simulink model "Target_Control_System"  (R2021b)
settings: Solver=FixedStepDiscrete  StartTime=0.0  StopTime=5  RelTol=1e-3
PreLoadFcn:
  | RTWConfigurationCB('preloadfcn', bdroot);
PostLoadFcn:
  | load('configuration/data_struct.mat');
  | load('configuration/fluxMaps_propMotor.mat');
  | load('configuration/parameterInit_PROP.mat');
  | load('configuration/parameterInit_PUMP.mat');
  | load('configuration/parameterInit_PITCH.mat');
  | load('configuration/parameterInit_TILT.mat');
  | %load('configuration/base_workspace_signal_definition.mat');
  | %load('resolvedatastores_to_baseworkspace_for_faster_simulation.mat');
model workspace (MAT data in the model file):
  SIMULATION_OPTIONS : Simulink.Parameter (value not decoded)
  TARGET_CODE_GEN : Simulink.Parameter (value not decoded)
  TCS_SAMPLE_FREQ_HZ : Simulink.Parameter (value not decoded)
symbols that are objects in the model workspace (value not decoded): TARGET_CODE_GEN, TCS_SAMPLE_FREQ_HZ
undefined symbols (not defined in the file): A_DQ_REF_LPF_INIT__PITCH, A_DQ_REF_LPF_INIT__PROP, A_DQ_REF_LPF_INIT__PUMP, A_DQ_REF_LPF_INIT__TILT, A_OBSERVER_CONFIDENCE_INIT__PITCH, A_OBSERVER_CONFIDENCE_INIT__PROP, A_OBSERVER_CONFIDENCE_INIT__PUMP, A_OBSERVER_CONFIDENCE_INIT__TILT, ACTUATOR_MAX_ANGLE_TRIP__PITCH, ACTUATOR_MIN_ANGLE_TRIP__PITCH, ACTUATOR_POS_SENSOR_INV_DIRECTION__PITCH, ACTUATOR_POS_SENSOR_INV_DIRECTION__TILT, ACTUATOR_POS_SENSOR_OFFSET__PITCH, ACTUATOR_POS_SENSOR_OFFSET__TILT, ADC_scaler1_baseaddr_TILT, ADC_SCALER_FLOAT_TO_FIXPOINT_EXPANSION, ANGLE_ELEC_FROM_SENSOR_OFFSET_INIT__PITCH, ANGLE_ELEC_FROM_SENSOR_OFFSET_INIT__PROP, ANGLE_ELEC_FROM_SENSOR_OFFSET_INIT__PUMP, ANGLE_ELEC_FROM_SENSOR_OFFSET_INIT__TILT, AUTO_CLEAR_FAULTS_ENABLED__PITCH, AUTO_CLEAR_FAULTS_ENABLED__PROP, AUTO_CLEAR_FAULTS_ENABLED__PUMP, AUTO_CLEAR_FAULTS_ENABLED__TILT, AUTO_CLEAR_FAULTS_WAIT_TICKS__PITCH, AUTO_CLEAR_FAULTS_WAIT_TICKS__PROP, AUTO_CLEAR_FAULTS_WAIT_TICKS__PUMP, AUTO_CLEAR_FAULTS_WAIT_TICKS__TILT, AUTO_I_ZERO_IDLE_TICKS__PITCH, AUTO_I_ZERO_IDLE_TICKS__PROP, AUTO_I_ZERO_IDLE_TICKS__PUMP, AUTO_I_ZERO_IDLE_TICKS__TILT, AUTO_I_ZERO_OFFSET_IDC_THRESHOLD__PITCH, AUTO_I_ZERO_OFFSET_IDC_THRESHOLD__PROP, AUTO_I_ZERO_OFFSET_IDC_THRESHOLD__PUMP, AUTO_I_ZERO_OFFSET_IDC_THRESHOLD__TILT, AUTO_I_ZERO_OFFSET_IPH_THRESHOLD__PITCH, AUTO_I_ZERO_OFFSET_IPH_THRESHOLD__PROP, AUTO_I_ZERO_OFFSET_IPH_THRESHOLD__PUMP, AUTO_I_ZERO_OFFSET_IPH_THRESHOLD__TILT, AUTO_SENSORLESS_SWITCHOVER_DISABLE_OMEGA, AUTO_SENSORLESS_SWITCHOVER_ENABLE_OMEGA, AUTO_SENSORLESS_SWITCHOVER_MIN_CONFIDENCE, AUXILIARY_PROTECTION_UNIT_BASEADDR__TILT, blanking_max_error_omega_INIT_PITCH, blanking_max_error_omega_INIT_TILT, blanking_max_error_position_INIT_PITCH, blanking_max_error_position_INIT_TILT, BRUTE_START_I_Q_REF_RAMP_SPEED__PITCH, BRUTE_START_I_Q_REF_RAMP_SPEED__PROP, BRUTE_START_I_Q_REF_RAMP_SPEED__PUMP, BRUTE_START_I_Q_REF_RAMP_SPEED__TILT, CONTROL_LOOP_DT_INIT__PITCH, CONTROL_LOOP_DT_INIT__PROP, CONTROL_LOOP_DT_INIT__PUMP, CONTROL_LOOP_DT_INIT__TILT, CORRECTION_FILTER_SCALE__PITCH, CORRECTION_FILTER_SCALE__PROP, CORRECTION_FILTER_SCALE__PUMP, CORRECTION_FILTER_SCALE__TILT ... (+458)
libraries: simulink x178, Reusables_Lib x24
(part 46 of 47)

== stateflow chart Target_Control_System/InterruptFunction/propMotor_isrTask/isrStateMachine/ISR State Machine ==
  state SuperState
    state ISR_States [parallel]
      // Main drive not active, just idle or various auxiliary operating modes
      // Do specific things:
      settings: executionOrder=3
      state Start
      state initiateCurrentOffsetNulling
        during:
        //Run an I controller for each current channel to be zerod, that zeros the actual reading
        // Note: the address to write out to
        oProp.oIsr_.oState_.fOffsetIntegratorIa_ += oProp.oIsr_.oIn_.oAdcData_.fIa_;
        oProp.oIsr_.oOut_.iOffsetIa_ -= cast((500.0F*oProp.oIsr_.oIn_.oAdcData_.fIa_ + 0.01F*oProp.oIsr_.oState_.fOffsetIntegratorIa_), int32);
        oProp.oIsr_.oState_.fOffsetIntegratorIb_ += oProp.oIsr_.oIn_.oAdcData_.fIb_;
        oProp.oIsr_.oOut_.iOffsetIb_ -= cast((500.0F*oProp.oIsr_.oIn_.oAdcData_.fIb_ + 0.01F*oProp.oIsr_.oState_.fOffsetIntegratorIb_), int32);
        oProp.oIsr_.oState_.fOffsetIntegratorIc_ += oProp.oIsr_.oIn_.oAdcData_.fIc_;
        oProp.oIsr_.oOut_.iOffsetIc_ -= cast((500.0F*oProp.oIsr_.oIn_.oAdcData_.fIc_ + 0.01F*oProp.oIsr_.oState_.fOffsetIntegratorIc_), int32);
        oProp.oIsr_.oState_.fOffsetIntegratorIdc_ += oProp.oIsr_.oIn_.oAdcData_.fIdc_;
        oProp.oIsr_.oOut_.iOffsetIdc_ -= cast((500.0F*oProp.oIsr_.oIn_.oAdcData_.fIdc_ + 0.01F*oProp.oIsr_.oState_.fOffsetIntegratorIdc_), int32);
        oProp.oIsr_.oOut_.iIBiasUpdated_ = 1;
      state CaptureAverageVoltage
        during:
        //At 50% duty, capture intended average phase voltage
        oProp.oIsr_.oState_.fOffsetAvgUphase_ += 0.001F * (oProp.oIsr_.oIn_.oAdcData_.fUdc_ * 0.5F - oProp.oIsr_.oState_.fOffsetAvgUphase_);
      state initiateVoltageOffsetNulling
        during:
        // At 50% duty, zero the voltage to the average voltage
        fTemp = oProp.oIsr_.oIn_.oAdcData_.fUa_ - oProp.oIsr_.oState_.fOffsetAvgUphase_;
        oProp.oIsr_.oState_.fOffsetIntegratorUa_ += fTemp;
        oProp.oIsr_.oOut_.iOffsetUa_ -= cast((50.0F * fTemp + 0.02F * oProp.oIsr_.oState_.fOffsetIntegratorUa_), int32);
        fTemp = oProp.oIsr_.oIn_.oAdcData_.fUb_ - oProp.oIsr_.oState_.fOffsetAvgUphase_;
        oProp.oIsr_.oState_.fOffsetIntegratorUb_ += fTemp;
        oProp.oIsr_.oOut_.iOffsetUb_ -= cast((50.0F * fTemp + 0.01F * oProp.oIsr_.oState_.fOffsetIntegratorUb_), int32);
        fTemp = oProp.oIsr_.oIn_.oAdcData_.fUc_ - oProp.oIsr_.oState_.fOffsetAvgUphase_;
        oProp.oIsr_.oState_.fOffsetIntegratorUc_ += fTemp;
        oProp.oIsr_.oOut_.iOffsetUc_ -= cast((50.0F * fTemp + 0.005F * oProp.oIsr_.oState_.fOffsetIntegratorUc_), int32);
        oProp.oIsr_.oOut_.iUBiasUpdated_ = 1;
      (default) -> Start
      Start -> initiateCurrentOffsetNulling [order 1] : [oProp.oIsr_.oIn_.uiDriveState_ == 95]
      initiateCurrentOffsetNulling -> Start : [!(oProp.oIsr_.oIn_.uiDriveState_ == 95)]
      Start -> CaptureAverageVoltage [order 2] : [oProp.oIsr_.oIn_.uiDriveState_ == 250 || oProp.oIsr_.oIn_.uiDriveState_ == 245]
      CaptureAverageVoltage -> Start : [!(oProp.oIsr_.oIn_.uiDriveState_ == 250 || oProp.oIsr_.oIn_.uiDriveState_ == 245)]
      Start -> initiateVoltageOffsetNulling [order 3] : [oProp.oIsr_.oIn_.uiDriveState_ == 251 || oProp.oIsr_.oIn_.uiDriveState_ == 246]
      initiateVoltageOffsetNulling -> Start : [!(oProp.oIsr_.oIn_.uiDriveState_ == 251 || oProp.oIsr_.oIn_.uiDriveState_ == 246)]
    state Software_overcurrent_protection [parallel]
      settings: executionOrder=2
      state Nominal
      state Fault
        state Fault_A
          entry:
          oProp.oMot_.oOut_.uiCurrentControllerActive_ = 0;
          oProp.oMot_.oOut_.uiEnableGateDrive_ = 0;
        state Fault_B
          // If we were already in a fault state, store the previous fault:
          entry:
          oProp.oMot_.oOut_.uiLastFaultState_ = oProp.oMot_.oState_.uiDriveState_;
        state Fault_C
          entry:
          oProp.oMot_.oState_.uiDriveState_ = 1007;
        (default) -> (junction 153)
        (junction 153) -> Fault_C [order 3]
        (junction 153) -> Fault_B [order 2] : [oProp.oMot_.oState_.uiDriveState_>= 1000]
        (junction 153) -> Fault_A [order 1] : [oProp.oMot_.oState_.uiDriveState_>= 200]
        Fault_A -> Fault_C [order 2]
        Fault_A -> Fault_B [order 1] : [oProp.oMot_.oState_.uiDriveState_>= 1000]
        Fault_B -> Fault_C
      (default) -> Nominal
      Fault -> Nominal : [oProp.oIsr_.oOut_.fIPhaseMagnitude_<oProp.oMot_.oParam_.fTripLimitSoftwareA_]
      Nominal -> Fault : [oProp.oIsr_.oOut_.fIPhaseMagnitude_>oProp.oMot_.oParam_.fTripLimitSoftwareA_]
    state Forced_Angle_State_Manager [parallel]
      settings: executionOrder=1
      state InitialForcedAngleState
        during:
        oProp.oMot_.oState_.oRampDataFluxMstrAngFrcd2clsdSmoothn_.fRampOut_ = 0.0F;
      state ForcedAngleState
        entry:
        oProp.oMot_.oOut_.uiForcedAngle_ = 1;
        during:
        oProp.oMot_.oState_.oRampDataFluxMstrAngFrcd2clsdSmoothn_.fRampOut_ = oProp.oIsr_.oState_.fFluxMasterAngle_ - oProp.oIsr_.oState_.fFluxMainAngleRaw2_;
      (default) -> InitialForcedAngleState
      InitialForcedAngleState -> ForcedAngleState : [oProp.oMot_.oState_.uiDriveState_ == 211 || oProp.oMot_.oState_.uiDriveState_ == 212]
      ForcedAngleState -> InitialForcedAngleState : [!(oProp.oMot_.oState_.uiDriveState_ == 211 || oProp.oMot_.oState_.uiDriveState_ == 212)]{oProp.oMot_.oOut_.uiForcedAngle_ = 0;}
  (default) -> SuperState
  data: oProp data_store_memory; fTemp local single

== stateflow chart Target_Control_System/InterruptFunction/pumpMotor_isrTask/isrStateMachine/ISR State Machine ==
  state SuperState
    state ISR_States [parallel]
      // Main drive not active, just idle or various auxiliary operating modes
      // Do specific things:
      settings: executionOrder=3
      state Start
      state initiateOffsetNulling
        during:
        //Run an I controller for each current channel to be zerod, that zeros the actual reading
        // Note: the address to write out to
        oPump.oIsr_.oState_.fOffsetIntegratorIa_ += oPump.oIsr_.oIn_.oAdcData_.fIa_;
        oPump.oIsr_.oOut_.iOffsetIa_ -= cast((500.0F*oPump.oIsr_.oIn_.oAdcData_.fIa_ + 0.01F*oPump.oIsr_.oState_.fOffsetIntegratorIa_), int32);
        oPump.oIsr_.oState_.fOffsetIntegratorIb_ += oPump.oIsr_.oIn_.oAdcData_.fIb_;
        oPump.oIsr_.oOut_.iOffsetIb_ -= cast((500.0F*oPump.oIsr_.oIn_.oAdcData_.fIb_ + 0.01F*oPump.oIsr_.oState_.fOffsetIntegratorIb_), int32);
        oPump.oIsr_.oState_.fOffsetIntegratorIc_ += oPump.oIsr_.oIn_.oAdcData_.fIc_;
        oPump.oIsr_.oOut_.iOffsetIc_ -= cast((500.0F*oPump.oIsr_.oIn_.oAdcData_.fIc_ + 0.01F*oPump.oIsr_.oState_.fOffsetIntegratorIc_), int32);
        oPump.oIsr_.oState_.fOffsetIntegratorIdc_ += oPump.oIsr_.oIn_.oAdcData_.fIdc_;
        oPump.oIsr_.oOut_.iOffsetIdc_ -= cast((500.0F*oPump.oIsr_.oIn_.oAdcData_.fIdc_ + 0.01F*oPump.oIsr_.oState_.fOffsetIntegratorIdc_), int32);
        oPump.oIsr_.oOut_.iIBiasUpdated_ = 1;
      (default) -> Start
      Start -> initiateOffsetNulling : [oPump.oMot_.oState_.uiDriveState_ == 95]
      initiateOffsetNulling -> Start : [!(oPump.oMot_.oState_.uiDriveState_ == 95)]
    state Forced_Angle_State_Manager [parallel]
      settings: executionOrder=1
      state InitialForcedAngleState
        during:
        oPump.oMot_.oState_.oRampDataFluxMstrAngFrcd2clsdSmoothn_.fRampOut_ = 0;
      state ForcedAngleState
        entry:
        oPump.oMot_.oOut_.uiForcedAngle_ = 1;
        during:
        oPump.oMot_.oState_.oRampDataFluxMstrAngFrcd2clsdSmoothn_.fRampOut_ = oPump.oIsr_.oState_.fFluxMasterAngle_ - oPump.oIsr_.oState_.fFluxMainAngleRaw2_;
      (default) -> InitialForcedAngleState
      InitialForcedAngleState -> ForcedAngleState : [oPump.oMot_.oState_.uiDriveState_ == 211 || oPump.oMot_.oState_.uiDriveState_ == 212]
      ForcedAngleState -> InitialForcedAngleState : [!(oPump.oMot_.oState_.uiDriveState_ == 211 || oPump.oMot_.oState_.uiDriveState_ == 212)]{oPump.oMot_.oOut_.uiForcedAngle_ = 0;}
    state Software_overcurrent_protection [parallel]
      settings: executionOrder=2
      state Nominal
      state Fault
        state Fault_A
          entry:
          oPump.oMot_.oOut_.uiCurrentControllerActive_ = 0;
          oPump.oMot_.oOut_.uiEnableGateDrive_ = 0;
        state Fault_B
          // If we were already in a fault state, store the previous fault:
          entry:
          oPump.oMot_.oOut_.uiLastFaultState_ = oPump.oMot_.oState_.uiDriveState_;
        state Fault_C
          entry:
          oPump.oMot_.oState_.uiDriveState_ = 1007;
        (default) -> (junction 153)
        (junction 153) -> Fault_C [order 3]
        (junction 153) -> Fault_B [order 2] : [oPump.oMot_.oState_.uiDriveState_>= 1000]
        (junction 153) -> Fault_A [order 1] : [oPump.oMot_.oState_.uiDriveState_>= 200]
        Fault_A -> Fault_C [order 2]
        Fault_A -> Fault_B [order 1] : [oPump.oMot_.oState_.uiDriveState_>= 1000]
        Fault_B -> Fault_C
      (default) -> Nominal
      Fault -> Nominal : [oPump.oIsr_.oOut_.fIPhaseMagnitude_<oPump.oMot_.oParam_.fTripLimitSoftwareA_]
      Nominal -> Fault : [oPump.oIsr_.oOut_.fIPhaseMagnitude_>oPump.oMot_.oParam_.fTripLimitSoftwareA_]
  (default) -> SuperState
  data: oPump data_store_memory

== stateflow chart Target_Control_System/InterruptFunction/tiltMotor_isrTask/isrStateMachine/ISR State Machine ==
  state SuperState
    state ISR_States [parallel]
      // Main drive not active, just idle or various auxiliary operating modes
      // Do specific things:
      settings: executionOrder=1
      state Start
      state initiateCurrentOffsetNulling
        during:
        //Run an I controller for each current channel to be zerod, that zeros the actual reading
        // Note: the address to write out to
        oTilt.oIsr_.oState_.fOffsetIntegratorIa_ += oTilt.oIsr_.oIn_.oAdcData_.fIa_;
        oTilt.oIsr_.oOut_.iOffsetIa_ -= cast((500.0F*oTilt.oIsr_.oIn_.oAdcData_.fIa_ + 0.01F*oTilt.oIsr_.oState_.fOffsetIntegratorIa_), int32);
        oTilt.oIsr_.oState_.fOffsetIntegratorIb_ += oTilt.oIsr_.oIn_.oAdcData_.fIb_;
        oTilt.oIsr_.oOut_.iOffsetIb_ -= cast((500.0F*oTilt.oIsr_.oIn_.oAdcData_.fIb_ + 0.01F*oTilt.oIsr_.oState_.fOffsetIntegratorIb_), int32);
        oTilt.oIsr_.oState_.fOffsetIntegratorIc_ += oTilt.oIsr_.oIn_.oAdcData_.fIc_;
        oTilt.oIsr_.oOut_.iOffsetIc_ -= cast((500.0F*oTilt.oIsr_.oIn_.oAdcData_.fIc_ + 0.01F*oTilt.oIsr_.oState_.fOffsetIntegratorIc_), int32);
        oTilt.oIsr_.oState_.fOffsetIntegratorIdc_ += oTilt.oIsr_.oIn_.oAdcData_.fIdc_;
        oTilt.oIsr_.oOut_.iOffsetIdc_ -= cast((500.0F*oTilt.oIsr_.oIn_.oAdcData_.fIdc_ + 0.01F*oTilt.oIsr_.oState_.fOffsetIntegratorIdc_), int32);
        oTilt.oIsr_.oOut_.iIBiasUpdated_ = 1;
      state CaptureAverageVoltage
        during:
        //At 50% duty, capture intended average phase voltage
        oTilt.oIsr_.oState_.fOffsetAvgUphase_ += 0.001F * (oTilt.oIsr_.oIn_.oAdcData_.fUdc_ * 0.5F - oTilt.oIsr_.oState_.fOffsetAvgUphase_);
      state initiateVoltageOffsetNulling
        during:
        // At 50% duty, zero the voltage to the average voltage
        fTemp = oTilt.oIsr_.oIn_.oAdcData_.fUa_ - oTilt.oIsr_.oState_.fOffsetAvgUphase_;
        oTilt.oIsr_.oState_.fOffsetIntegratorUa_ += fTemp;
        oTilt.oIsr_.oOut_.iOffsetUa_ -= cast((50.0F * fTemp + 0.02F * oTilt.oIsr_.oState_.fOffsetIntegratorUa_), int32);
        fTemp = oTilt.oIsr_.oIn_.oAdcData_.fUb_ - oTilt.oIsr_.oState_.fOffsetAvgUphase_;
        oTilt.oIsr_.oState_.fOffsetIntegratorUb_ += fTemp;
        oTilt.oIsr_.oOut_.iOffsetUb_ -= cast((50.0F * fTemp + 0.01F * oTilt.oIsr_.oState_.fOffsetIntegratorUb_), int32);
        fTemp = oTilt.oIsr_.oIn_.oAdcData_.fUc_ - oTilt.oIsr_.oState_.fOffsetAvgUphase_;
        oTilt.oIsr_.oState_.fOffsetIntegratorUc_ += fTemp;
        oTilt.oIsr_.oOut_.iOffsetUc_ -= cast((50.0F * fTemp + 0.005F * oTilt.oIsr_.oState_.fOffsetIntegratorUc_), int32);
        oTilt.oIsr_.oOut_.iUBiasUpdated_ = 1;
      (default) -> Start
      Start -> initiateCurrentOffsetNulling [order 1] : [oTilt.oIsr_.oIn_.uiDriveState_ == 95]
      initiateCurrentOffsetNulling -> Start : [!(oTilt.oIsr_.oIn_.uiDriveState_ == 95)]
      Start -> CaptureAverageVoltage [order 2] : [oTilt.oIsr_.oIn_.uiDriveState_ == 250 || oTilt.oIsr_.oIn_.uiDriveState_ == 245]
      CaptureAverageVoltage -> Start : [!(oTilt.oIsr_.oIn_.uiDriveState_ == 250 || oTilt.oIsr_.oIn_.uiDriveState_ == 245)]
      Start -> initiateVoltageOffsetNulling [order 3] : [oTilt.oIsr_.oIn_.uiDriveState_ == 251 || oTilt.oIsr_.oIn_.uiDriveState_ == 246]
      initiateVoltageOffsetNulling -> Start : [!(oTilt.oIsr_.oIn_.uiDriveState_ == 251 || oTilt.oIsr_.oIn_.uiDriveState_ == 246)]
  (default) -> SuperState
  data: oTilt data_store_memory; fTemp local single

== stateflow chart Target_Control_System/MainLoop/tiltMotor_mainLoop/Decimation gate for 200 Hz Tilt/motorTaskMainDecimationAStep(&oTilt)/Check zero current if inverter off/Enabled Subsystem/Chart ==
  state Start
  state Drive_trip
    // Disable the drive and enter a trip state (error state)
    entry:
    oTilt.oMot_.oOut_.uiEnableGateDrive_ = 0;
    oTilt.oMot_.oOut_.uiCurrentControllerActive_ = 0;
    // NOTE: the actual turning off is done in the ctrl interrupt
    // formerly: Xil_Out32(uiGateDriverBaseaddr_, 0x0);
  state Store_previous_fault
    // If we were already in a fault state, store the previous fault:
    entry:
    oTilt.oMot_.oOut_.uiLastFaultState_ = oTilt.oMot_.oState_.uiDriveState_;
  state setTripState
    entry:
    oTilt.oMot_.oState_.uiDriveState_ = 1042;
  (default) -> Start
  setTripState -> Start
  Start -> (junction 14) : [fabs(oTilt.oMot_.oIn_.oAdcData_.fIa_) > oTilt.oMot_.oParam_.fMaximumPhaseCurrentWhileOff_ || ...
      | fabs(oTilt.oMot_.oIn_.oAdcData_.fIb_) > oTilt.oMot_.oParam_.fMaximumPhaseCurrentWhileOff_ || ...
      | fabs(oTilt.oMot_.oIn_.oAdcData_.fIc_) > oTilt.oMot_.oParam_.fMaximumPhaseCurrentWhileOff_]
  (junction 14) -> Drive_trip [order 1] : [oTilt.oMot_.oState_.uiDriveState_ >= 200]
  (junction 14) -> (junction 19) [order 2]
  Drive_trip -> (junction 19)
  (junction 19) -> Store_previous_fault [order 1] : [oTilt.oMot_.oState_.uiDriveState_ >= 1000]
  (junction 19) -> setTripState [order 2]
  Store_previous_fault -> setTripState
  data: oTilt data_store_memory

== stateflow chart Target_Control_System/MainLoop/propMotor_mainLoop/motorStateMachineLogic(&oProp)/Idle-Loop State Machine Prop ==
  state motorStateMachineLogic
  state State_90
    //startup delay
    state Wait_Ticks_
    state Startup_Delay_
      entry:
      oProp.oMot_.oState_.uiDriveState_ = 95;
      oProp.oMot_.oOut_.uiLastFaultState_ = 0;
    (default) -> State_90.Wait_Ticks_
    State_90.Wait_Ticks_ -> Startup_Delay_ : [after(35, tick)]
  state State_246
    // Second phase of voltage nulling
    state Wait_uiDelayTicks_
    state Next
      entry:
      oProp.oMot_.oState_.uiDriveState_ = 100;
      oProp.oMot_.oOut_.uiEnableGateDrive_ = 0x0;
      oProp.oMot_.oIn_.uiVoltageOffsetNullingActive_ = 0;
    (default) -> State_246.Wait_uiDelayTicks_
    State_246.Wait_uiDelayTicks_ -> State_246.Next : [after(25, tick)]
  state State_95
    // Current offset nulling
    state Wait_Ticks_
    state Current_offset_nulling
      entry:
      oProp.oMot_.oState_.uiCurrentOffsetNullingPerformed_++;
      oProp.oMot_.oIn_.uiCurrentOffsetNullingActive_ = 0;
      oProp.oMot_.oIn_.uiVoltageOffsetNullingActive_ = 0;
      oProp.oMot_.oState_.uiDriveState_ = 99;
      //SZ: still need to re-write the FPGA protection to enable the sum of current detection for fault 1034
    (default) -> State_95.Wait_Ticks_
    State_95.Wait_Ticks_ -> Current_offset_nulling : [after(6, tick)]
  state State_245
    // Initial phase of voltage nulling
    state Wait_uiDelayTicks_
    state Next
      entry:
      oProp.oMot_.oState_.uiDriveState_ = 246;
    (default) -> State_245.Wait_uiDelayTicks_
    State_245.Wait_uiDelayTicks_ -> State_245.Next : [after(25, tick)]
  state State_99
    // Minimum command set not met. Also the return state after clearing trips etc.
    state Substate
    state Idle_state
      entry:
      oProp.oMot_.oState_.uiDriveState_ = 100;
    state Cleanup
      // We somehow left the forced angle start sequence without cleaning up.
      // Clean up now.
      entry:
      oProp.oMot_.oState_.oRampDataOmegaERef_.oParam_.fUpslope_ = oProp.oMot_.oState_.fForcedAngleStartOrigOmegaRamp_;
      oProp.oMot_.oState_.oRampDataOmegaERef_.fSetpoint_ = fabs(oProp.oMot_.oState_.fForcedAngleStartOrigOmega_);
      oProp.oMot_.oState_.uiSpeedControllerActive_ = oProp.oMot_.oState_.uiForcedAngleStartOrigSpeedControllerActive_;
      oProp.oMot_.oState_.oRampDataIqRef_.oParam_.fUpslope_ = oProp.oMot_.oState_.fForcedAngleStartOrigIRamp_;
      oProp.oMot_.oState_.oRampDataIqRef_.oParam_.fDownslope_ = oProp.oMot_.oState_.oRampDataIqRef_.oParam_.fUpslope_;
      oProp.oMot_.oOut_.uiForcedAngle_ = 0;
      oProp.oMot_.oState_.uiForcedAngleStartParametersSet_ = 0;
    (default) -> State_99.Substate
    State_99.Substate -> (junction 218)
    (junction 218) -> Idle_state [order 2] : [!oProp.oMot_.oState_.uiMinimumCommandSetFlags_]
    (junction 218) -> State_99.Cleanup [order 1] : [oProp.oMot_.oState_.uiForcedAngleStartParametersSet_]
    State_99.Cleanup -> Idle_state : [!oProp.oMot_.oState_.uiMinimumCommandSetFlags_]
  state State_104
    // Idle, motor spinning (windmilling, coasting down),
    // autostart enabled, and a nonzero current applied
    // Removed autostart functionality
    entry:
    oProp.oMot_.oState_.uiDriveState_ = 102;
  state State_103
    // Idle, motor not spinning, autostart enabled, and a nonzero current applied
    // Removed autostart functionality
    entry:
    oProp.oMot_.oState_.uiDriveState_ = 101;
  state State_100
    //Idle, determine if the motor is externally driven (e.g. windmilling or spindown) or standing still
    state Initialization
      entry:
      oProp.oMot_.oState_.oRampDataOmegaERef_.fRampOut_ = 0.0;
      oProp.oMot_.oState_.oRampDataIqRef_.fRampOut_ = 0.0;
    state Entering_State_101
      entry:
      oProp.oMot_.oState_.uiDriveState_ = 101;
    state Cleanup
      // We somehow left the forced angle start sequence without cleaning up.
      // Clean up now.
      entry:
      oProp.oMot_.oState_.uiDriveState_  = 99;
    state Entering_State_102
      entry:
      oProp.oMot_.oState_.uiDriveState_ = 102;
    state pwm50PercentDuty
      //Pre-set 50% duty
      entry:
      oProp.oMot_.oOut_.uiPwmRequestFromMain_ = 1;
      oProp.oMot_.oOut_.uiPwmDutyTicksFromMainA_ = cast(((oProp.oMot_.oParam_.fPwmPeriodTicksMainloopFloat_) / 2), uint32);
      oProp.oMot_.oOut_.uiPwmDutyTicksFromMainB_ = cast(((oProp.oMot_.oParam_.fPwmPeriodTicksMainloopFloat_) / 2), uint32);
      oProp.oMot_.oOut_.uiPwmDutyTicksFromMainC_ = cast(((oProp.oMot_.oParam_.fPwmPeriodTicksMainloopFloat_) / 2), uint32);
    (default) -> State_100.Initialization
    State_100.Initialization -> (junction 235)
    (junction 235) -> (junction 251) [order 2]
    (junction 251) -> Entering_State_101 [order 1] : [(fabs(oProp.oMot_.oOut_.fOmegaEObserverXlpf2_) < oProp.oMot_.oParam_.fFlyingStartOmegaELimit_) ....
        |  || (oProp.oMot_.oState_.fObserverConfidence_ < 0.7F)]
    (junction 235) -> State_100.Cleanup [order 1] : [oProp.oMot_.oState_.uiMinimumCommandSetFlags_]
    (junction 251) -> Entering_State_102 [order 2]
    Entering_State_101 -> pwm50PercentDuty
    Entering_State_102 -> pwm50PercentDuty
  state State_224
    state Transition_220
      // Direction or confidence check failed, restart full sequence
      entry:
      oProp.oMot_.oState_.uiDriveState_ = 220;
    state FlyingStart
      entry:
      oProp.oMot_.oOut_.uiPwmDutyTicksFromMainA_ = uint32((oProp.oMot_.oParam_.fPwmPeriodTicksMainloopFloat_)/2);
      oProp.oMot_.oOut_.uiPwmDutyTicksFromMainB_ = uint32((oProp.oMot_.oParam_.fPwmPeriodTicksMainloopFloat_)/2);
      oProp.oMot_.oOut_.uiPwmDutyTicksFromMainC_ = uint32((oProp.oMot_.oParam_.fPwmPeriodTicksMainloopFloat_)/2);
      oProp.oMot_.oState_.oRampDataOmegaERef_.fRampOut_ = oProp.oMot_.oIn_.fOmegaEObserverLpf2_;
      oProp.oMot_.oState_.oRampDataIqRef_.fRampOut_ = 0.0;
      oProp.oIsr_.oParam_.oPiDataIq_.fState_ = 0.0F;
      oProp.oIsr_.oParam_.oPiDataId_.fState_ = 0.0F;
      oProp.oMot_.oParam_.oPiDataRpm_.fState_ = 0.0F;
      oProp.oMot_.oParam_.oPid2DataRpmCtrl_.fState_ = 0.0F;
      oProp.oMot_.oState_.uiDriveState_ = 200;
      // release gate signals
      oProp.oMot_.oOut_.uiEnableGateDrive_ = 0x7;
      // Release control in main interrupt
      oProp.oMot_.oOut_.uiCurrentControllerActive_ = 1;
    state uiAutomaticFanControlMode_
      entry:
      oProp.oMot_.oState_.uiDriveState_ = 205;
    (default) -> (junction 543)
    (junction 543) -> (junction 546) [order 2]
    (junction 543) -> (junction 545) [order 1] : [oProp.oMot_.oState_.fObserverConfidence_ > oProp.oMot_.oParam_.fSlaveStartMinConfidence_ && ....
        | !(oProp.oMot_.oOut_.fOmegaEObserverXlpf2_ * oProp.oMot_.oState_.fForcedAngleStartDirection_ < 0.0F)]
        | // The faster we go, the further we jump in the sequence
        | // [SZ]: need to investigate implementing the __signbitf() function in Stateflow]
    (junction 546) -> State_224.Transition_220
    (junction 545) -> FlyingStart : //Confidence wise we're good to go, but is the speed high enough?
        | [fabs(oProp.oMot_.oOut_.fOmegaEObserverXlpf2_) > ....
        |  (oProp.oMot_.oParam_.fSlaveStartMinOmegaE_)]
    FlyingStart -> State_224.uiAutomaticFanControlMode_ : [oProp.oMot_.oParam_.uiAutomaticFanControlMode_ == 1]
  state State_102
    // Idle, motor spinning by external means (windmilling, downhill, large inertia, ....)
    state Stay_at_102
      entry:
      oProp.oMot_.oState_.uiDriveState_ = 102;
    state Transition_to_101
      entry:
      oProp.oMot_.oState_.uiDriveState_ = 101;
    (default) -> (junction 349)
    (junction 349) -> Stay_at_102 [order 2]
    (junction 349) -> Transition_to_101 [order 1] : [fabs(oProp.oMot_.oOut_.fOmegaEObserverXlpf2_) < oProp.oMot_.oParam_.fFlyingStartOmegaELimit_ ....
        | || oProp.oMot_.oState_.fObserverConfidence_ < 0.65F]
  state State_222
    state Transition_224
      entry:
      oProp.oMot_.oState_.uiDriveState_ = 224;
    state Transition_223
      entry:
      oProp.oMot_.oState_.uiDriveState_ = 223;
    state Transition_220
      // Direction or confidence check failed, restart full sequence
      entry:
      oProp.oMot_.oState_.uiDriveState_ = 220;
    (default) -> (junction 521)
    (junction 521) -> (junction 518) [order 2]
    (junction 521) -> (junction 512) [order 1] : [oProp.oMot_.oState_.fObserverConfidence_ > oProp.oMot_.oParam_.fSlaveStartMinConfidence_ && ....
        | !(oProp.oMot_.oOut_.fOmegaEObserverXlpf2_ * oProp.oMot_.oState_.fForcedAngleStartDirection_ < 0.0F)]
        | // The faster we go, the further we jump in the sequence
        | // [SZ]: need to investigate implementing the __signbitf() function in Stateflow]
    (junction 518) -> State_222.Transition_220
    (junction 512) -> (junction 519) [order 1]
    (junction 519) -> State_222.Transition_224 : [fabs(oProp.oMot_.oOut_.fOmegaEObserverXlpf2_) >....
        |  (oProp.oMot_.oParam_.fSlaveStartMinOmegaE_)]
    (junction 512) -> State_222.Transition_223 [order 2]
  state State_223
    state Transition_220
      // Direction or confidence check failed, restart full sequence
      entry:
      oProp.oMot_.oState_.uiDriveState_ = 220;
    state Transition_224
      entry:
      oProp.oMot_.oState_.uiDriveState_ = 224;
    (default) -> (junction 528)
    (junction 528) -> (junction 524) [order 2]
    (junction 528) -> (junction 533) [order 1] : [oProp.oMot_.oState_.fObserverConfidence_ > oProp.oMot_.oParam_.fSlaveStartMinConfidence_ && ....
        | !(oProp.oMot_.oOut_.fOmegaEObserverXlpf2_ * oProp.oMot_.oState_.fForcedAngleStartDirection_ < 0.0F)]
        | // The faster we go, the further we jump in the sequence
        | // [SZ]: need to investigate implementing the __signbitf() function in Stateflow]
    (junction 524) -> State_223.Transition_220
    (junction 533) -> State_223.Transition_224 : [fabs( oProp.oMot_.oOut_.fOmegaEObserverXlpf2_) >....
        |  (oProp.oMot_.oParam_.fSlaveStartMinOmegaE_)]
  state State_101
    // Idle, motor not spinning
    state Initialization
      entry:
      oProp.oMot_.oState_.oRampDataOmegaERef_.fRampOut_ = 0.0;
      oProp.oMot_.oState_.oRampDataIqRef_.fRampOut_ = 0.0;
    state Transition_to_102
      entry:
      oProp.oMot_.oState_.uiDriveState_ = 102;
    (default) -> State_101.Initialization
    State_101.Initialization -> (junction 340)
    (junction 340) -> Transition_to_102 [order 1] : [(fabs(oProp.oMot_.oOut_.fOmegaEObserverXlpf2_) > oProp.oMot_.oParam_.fFlyingStartOmegaELimit_) ....
        | && (oProp.oMot_.oState_.fObserverConfidence_ > 0.65F)]
  state State_220
    // Flying start, first of multiple stages.
    // There has to be an uninterrupted chain of OKs. Too low confidence at any step,
    // and fall back to this initial state.
    state Substate
    state Transition_224
      entry:
      oProp.oMot_.oState_.uiDriveState_ = 224;
    state Transition_223
      entry:
      oProp.oMot_.oState_.uiDriveState_ = 223;
    state Transition_222
      entry:
      oProp.oMot_.oState_.uiDriveState_ = 222;
    state Transition_221
      /* Don't check for the speed for the slowest
      //advancement path, that will happen in state 224 */
      entry:
      oProp.oMot_.oState_.uiDriveState_ = 221;
    (default) -> State_220.Substate
    State_220.Substate -> (junction 443)
    (junction 443) -> (junction 396) : [oProp.oMot_.oState_.fObserverConfidence_ > oProp.oMot_.oParam_.fSlaveStartMinConfidence_ && ....
        | !(oProp.oMot_.oOut_.fOmegaEObserverXlpf2_ * oProp.oMot_.oState_.fForcedAngleStartDirection_ < 0.0F)]
        | // The faster we go, the further we jump in the sequence
        | // [SZ]: need to investigate implementing the __signbitf() function in Stateflow]
    (junction 396) -> (junction 422) [order 1]
    (junction 396) -> (junction 430) [order 3]
    (junction 430) -> (junction 435) [order 2]
    (junction 422) -> State_220.Transition_224 : [fabs(oProp.oMot_.oOut_.fOmegaEObserverXlpf2_) >....
        |  (oProp.oMot_.oParam_.fSlaveStartMinOmegaE_)]
    (junction 396) -> State_220.Transition_223 [order 2] : [fabs(4.0F * oProp.oMot_.oOut_.fOmegaEObserverXlpf2_) >....
        |  (3.0F * oProp.oMot_.oParam_.fSlaveStartMinOmegaE_)]
    (junction 430) -> State_220.Transition_222 [order 1] : [fabs(2.0F*oProp.oMot_.oOut_.fOmegaEObserverXlpf2_) >....
        |  (oProp.oMot_.oParam_.fSlaveStartMinOmegaE_)]
    (junction 435) -> Transition_221
  state State_221
    state Transition_224
      entry:
      oProp.oMot_.oState_.uiDriveState_ = 224;
    state Transition_223
      entry:
      oProp.oMot_.oState_.uiDriveState_ = 223;
    state Transition_222
      entry:
      oProp.oMot_.oState_.uiDriveState_ = 222;
    state Transition_220
      // Direction or confidence check failed, restart full sequence
      entry:
      oProp.oMot_.oState_.uiDriveState_ = 220;
    (default) -> (junction 453)
    (junction 453) -> (junction 450) [order 2]
    (junction 453) -> (junction 459) [order 1] : [oProp.oMot_.oState_.fObserverConfidence_ > oProp.oMot_.oParam_.fSlaveStartMinConfidence_ && ....
        | !(oProp.oMot_.oOut_.fOmegaEObserverXlpf2_ * oProp.oMot_.oState_.fForcedAngleStartDirection_ < 0.0F)]
        | // The faster we go, the further we jump in the sequence
        | // [SZ]: need to investigate implementing the __signbitf() function in Stateflow]
    (junction 450) -> State_221.Transition_220
    (junction 459) -> (junction 461) [order 1]
    (junction 459) -> (junction 451) [order 3]
    (junction 461) -> State_221.Transition_224 : [fabs(oProp.oMot_.oOut_.fOmegaEObserverXlpf2_) >....
        |  (oProp.oMot_.oParam_.fSlaveStartMinOmegaE_)]
    (junction 459) -> State_221.Transition_223 [order 2] : [fabs(4.0F * oProp.oMot_.oOut_.fOmegaEObserverXlpf2_) >....
        |  (3.0F * oProp.oMot_.oParam_.fSlaveStartMinOmegaE_)]
    (junction 451) -> State_221.Transition_222
  state State_212
    // Forced angle. Current and speed are ramping.
    // Once we reach a certain predefined speed, turn off forced angle
    // (idea: look at observer confidence instead, or additionally)
    state Wait_RPM
      exit:
      // To avoid a sudden step in angle, add an offset to the estimated angle to give the forced angle. It'll ramp to zero
      //oProp.oMot_.oState_.oRampDataFluxMstrAngFrcd2clsdSmoothn_.fRampOut_ = oProp.oIsr_.oState_.fFluxMasterAngle_ - oProp.oIsr_.oState_.fFluxMainAngleRaw2_;
    state Restore_values
      // Restore values: (Mind the order of setting things, in case the interrupt starts halfway through)
      state Reset
        entry:
        oProp.oMot_.oOut_.uiForcedAngle_ = 0;
        oProp.oMot_.oState_.oRampDataOmegaERef_.oParam_.fUpslope_ = oProp.oMot_.oState_.fForcedAngleStartOrigOmegaRamp_;
        // The downslope wasn't touched in the first place, as forced angle start only relies on the upslope
        oProp.oMot_.oState_.uiDriveState_ = 213;
      (default) -> (junction 79)
      (junction 79) -> (junction 586) [order 1] : [oProp.oMot_.oState_.oRampDataFluxMstrAngFrcd2clsdSmoothn_.fRampOut_> PI_F]
          | {oProp.oMot_.oState_.oRampDataFluxMstrAngFrcd2clsdSmoothn_.fRampOut_ -= TWO_PI_F;}
      (junction 586) -> Reset [order 2]
      (junction 79) -> Reset [order 3]
      (junction 79) -> Reset [order 2] : [oProp.oMot_.oState_.oRampDataFluxMstrAngFrcd2clsdSmoothn_.fRampOut_ < -PI_F]
          | {oProp.oMot_.oState_.oRampDataFluxMstrAngFrcd2clsdSmoothn_.fRampOut_ += TWO_PI_F;}
      (junction 586) -> Reset [order 1] : [oProp.oMot_.oState_.oRampDataFluxMstrAngFrcd2clsdSmoothn_.fRampOut_ < -PI_F]
          | {oProp.oMot_.oState_.oRampDataFluxMstrAngFrcd2clsdSmoothn_.fRampOut_ += TWO_PI_F;}
    (default) -> Wait_RPM
    Wait_RPM -> Restore_values : [oProp.oMot_.oState_.oRampDataOmegaERef_.fRampOut_ > oProp.oMot_.oParam_.fForcedAngleOmegaEHandoff_ ]
  state State_213
    // Almost the end of forced angle
    state Wait_uiForcedStartPostTicks_
      exit:
      oProp.oMot_.oState_.oRampDataIqRef_.oParam_.fUpslope_ = oProp.oMot_.oState_.fForcedAngleStartOrigIRamp_;	// TODO whatabout downslope
      oProp.oMot_.oState_.oRampDataIqRef_.oParam_.fDownslope_ = oProp.oMot_.oState_.oRampDataIqRef_.oParam_.fUpslope_;
      oProp.oMot_.oState_.uiForcedAngleStartParametersSet_ = 0;
      oProp.oMot_.oState_.uiDriveState_ = 200;
    state uiAutomaticFanControlMode_
      entry:
      oProp.oMot_.oState_.uiDriveState_ = 205;
    (default) -> Wait_uiForcedStartPostTicks_
    Wait_uiForcedStartPostTicks_ -> (junction 584) : [after(oProp.oMot_.oParam_.uiForcedStartPostTicks_, tick)]
    (junction 584) -> (junction 576) [order 2]
    (junction 584) -> State_213.uiAutomaticFanControlMode_ [order 1] : [oProp.oMot_.oParam_.uiAutomaticFanControlMode_ == 1]
    State_213.uiAutomaticFanControlMode_ -> (junction 576)
  state State_211
    // Forced angle start, ramping the current while holding speed at zero.
    // After some time, we release the speed
    state Wait_uiForcedAngleSpeedDelayTicks_
    state Speed_loop_active
      entry:
      oProp.oMot_.oState_.oRampDataOmegaERef_.fSetpoint_ = oProp.oMot_.oState_.fForcedAngleStartOrigOmega_;
    state Speed_loop_inactive
      // Torque control. We don't actually know if the current is enough to reach the handoff point
      // So, we set the speedref to a bit above the handoff point. Past the handoff, this value becomes irrelevant.
      entry:
      oProp.oMot_.oState_.oRampDataOmegaERef_.fSetpoint_ = oProp.oMot_.oParam_.fForcedAngleOmegaEHandoff_ * 1.1F;
    state Bidirection
      // allow for clock and counterclockwise dir depending on current setpoint
      entry:
      oProp.oMot_.oState_.oRampDataOmegaERef_.fSetpoint_ = abs(oProp.oMot_.oState_.oRampDataOmegaERef_.fSetpoint_) * oProp.oMot_.oState_.fForcedAngleStartDirection_;
      oProp.oMot_.oState_.uiDriveState_ = 212;
    (default) -> Wait_uiForcedAngleSpeedDelayTicks_
    Wait_uiForcedAngleSpeedDelayTicks_ -> (junction 60) : [after(oProp.oMot_.oParam_.uiForcedAngleSpeedDelayTicks_, tick)]
    (junction 60) -> Speed_loop_active [order 1] : [oProp.oMot_.oState_.uiSpeedControllerActive_ == 1]
    (junction 60) -> Speed_loop_inactive [order 2]
    Speed_loop_active -> Bidirection
    Speed_loop_inactive -> Bidirection
  (default) -> motorStateMachineLogic
  motorStateMachineLogic -> State_90 [order 1] : [oProp.oMot_.oState_.uiDriveState_ == 90]
  State_90 -> motorStateMachineLogic : [!(oProp.oMot_.oState_.uiDriveState_ == 90)]
  motorStateMachineLogic -> State_246 [order 12] : [oProp.oMot_.oState_.uiDriveState_ == 246]
  State_246 -> motorStateMachineLogic : [!(oProp.oMot_.oState_.uiDriveState_ == 246)]
  motorStateMachineLogic -> State_95 [order 2] : [oProp.oMot_.oState_.uiDriveState_ == 95]
  Current_offset_nulling -> motorStateMachineLogic : [!(oProp.oMot_.oState_.uiDriveState_ == 95)]
  motorStateMachineLogic -> State_245 [order 11] : [oProp.oMot_.oState_.uiDriveState_ == 245]
  State_245 -> motorStateMachineLogic : [!(oProp.oMot_.oState_.uiDriveState_ == 245)]
  motorStateMachineLogic -> State_99 [order 3] : [oProp.oMot_.oState_.uiDriveState_ == 99]
  State_99 -> motorStateMachineLogic : [!(oProp.oMot_.oState_.uiDriveState_ == 99)]
  motorStateMachineLogic -> State_104 [order 8] : [oProp.oMot_.oState_.uiDriveState_ == 104]
  State_104 -> motorStateMachineLogic
  motorStateMachineLogic -> State_103 [order 7] : [oProp.oMot_.oState_.uiDriveState_ == 103]
  State_103 -> motorStateMachineLogic
  motorStateMachineLogic -> State_100 [order 4] : [oProp.oMot_.oState_.uiDriveState_ == 100]
  motorStateMachineLogic -> State_102 [order 6] : [oProp.oMot_.oState_.uiDriveState_ == 102]
  Stay_at_102 -> motorStateMachineLogic
  State_100.Cleanup -> motorStateMachineLogic
  Transition_to_101 -> motorStateMachineLogic
  pwm50PercentDuty -> motorStateMachineLogic
  motorStateMachineLogic -> State_101 [order 5] : [oProp.oMot_.oState_.uiDriveState_ == 101]
  (junction 340) -> motorStateMachineLogic [order 2] : // We're staying at rest.
  Transition_to_102 -> motorStateMachineLogic
  State_224 -> (junction 417) : [!(oProp.oMot_.oState_.uiDriveState_ == 224)]
  (junction 417) -> State_224 [order 4] : [oProp.oMot_.oState_.uiDriveState_ == 224]
  State_223 -> (junction 417) : [!(oProp.oMot_.oState_.uiDriveState_ == 223)]
  (junction 417) -> State_223 [order 3] : [oProp.oMot_.oState_.uiDriveState_ == 223]
  State_222 -> (junction 417) : [!(oProp.oMot_.oState_.uiDriveState_ == 222)]
  (junction 439) -> State_222 [order 2] : [oProp.oMot_.oState_.uiDriveState_ == 222]
  (junction 417) -> motorStateMachineLogic [order 5]
  motorStateMachineLogic -> (junction 417) [order 10] : [(oProp.oMot_.oState_.uiDriveState_ >= 220) && (oProp.oMot_.oState_.uiDriveState_ <= 224) ]
  (junction 417) -> (junction 439) [order 2]
  State_221 -> (junction 417) : [!(oProp.oMot_.oState_.uiDriveState_ == 221)]
  State_220 -> (junction 417) : [!(oProp.oMot_.oState_.uiDriveState_ == 220)]
  (junction 417) -> State_220 [order 1] : [oProp.oMot_.oState_.uiDriveState_ == 220]
  (junction 439) -> State_221 [order 1] : [oProp.oMot_.oState_.uiDriveState_ == 221]
  motorStateMachineLogic -> (junction 560) [order 9] : [oProp.oMot_.oState_.uiDriveState_ == 211]
  (junction 560) -> motorStateMachineLogic [order 4]
  (junction 576) -> (junction 560) : {oProp.oMot_.oState_.oRampDataIqRef_.oParam_.fUpslope_ = oProp.oMot_.oState_.fForcedAngleStartOrigIRamp_;
      |  oProp.oMot_.oState_.oRampDataIqRef_.oParam_.fDownslope_ = oProp.oMot_.oState_.oRampDataIqRef_.oParam_.fUpslope_;
      |  oProp.oMot_.oState_.uiForcedAngleStartParametersSet_ = 0;}
  State_212 -> (junction 560) : [!(oProp.oMot_.oState_.uiDriveState_ == 212)]
      | {oProp.oMot_.oState_.oRampDataOmegaERef_.oParam_.fUpslope_ = oProp.oMot_.oState_.fForcedAngleStartOrigOmegaRamp_;
      | oProp.oMot_.oState_.oRampDataOmegaERef_.fSetpoint_ = fabs(oProp.oMot_.oState_.fForcedAngleStartOrigOmega_);
      | oProp.oMot_.oState_.oRampDataOmegaERef_.fRampOut_ = oProp.oMot_.oOut_.fOmegaEObserverXlpf2_;  // For the speed controller, if used
      | oProp.oMot_.oState_.uiSpeedControllerActive_ = oProp.oMot_.oState_.uiForcedAngleStartOrigSpeedControllerActive_;
      | oProp.oMot_.oOut_.uiForcedAngle_ = 0;}
  (junction 560) -> State_212 [order 2] : [oProp.oMot_.oState_.uiDriveState_ == 212]
  (junction 560) -> State_213 [order 3] : [oProp.oMot_.oState_.uiDriveState_ == 213]
  State_211 -> (junction 560) : [!(oProp.oMot_.oState_.uiDriveState_ == 211)]
  (junction 560) -> State_211 [order 1] : [oProp.oMot_.oState_.uiDriveState_ == 211]
  data: oProp data_store_memory; PI_F constant single =3.14159265359; TWO_PI_F constant single =6.28318530718

== stateflow chart Target_Control_System/InterruptFunction/allMotors_readAdc/Sensor Offset Calibration VP ==
  state SuperState
    state Calibrate_PhaseCurrent [parallel]
      settings: executionOrder=1
      state EnabledDontCalibrate
      state Average
        during:
        oPitch.oIsr_.oState_.fOffsetIntegratorIa_ += oPitch.oIsr_.oIn_.oAdcData_.fIa_;
        oPitch.oIsr_.oOut_.iOffsetIa_ -= cast((500.0F*oPitch.oIsr_.oIn_.oAdcData_.fIa_ + 0.01F*oPitch.oIsr_.oState_.fOffsetIntegratorIa_), int32);
        oPitch.oIsr_.oState_.fOffsetIntegratorIb_ += oPitch.oIsr_.oIn_.oAdcData_.fIb_;
        oPitch.oIsr_.oOut_.iOffsetIb_ -= cast((500.0F*oPitch.oIsr_.oIn_.oAdcData_.fIb_ + 0.01F*oPitch.oIsr_.oState_.fOffsetIntegratorIb_), int32);
        oPitch.oIsr_.oState_.fOffsetIntegratorIc_ += oPitch.oIsr_.oIn_.oAdcData_.fIc_;
        oPitch.oIsr_.oOut_.iOffsetIc_ -= cast((500.0F*oPitch.oIsr_.oIn_.oAdcData_.fIc_ + 0.01F*oPitch.oIsr_.oState_.fOffsetIntegratorIc_), int32);
        oPitch.oIsr_.oOut_.iIBiasUpdated_ = 1;
      state Finish
      (default) -> EnabledDontCalibrate
      EnabledDontCalibrate -> Average : [oPitch.oMot_.oOut_.uiEnable_ == 0]
      Average -> Finish : [oPitch.oMot_.oOut_.uiEnable_  == 1 || after(0.6*80000, tick)]
  data: oPitch data_store_memory

== stateflow chart Target_Control_System/MainLoop/propMotor_mainLoop/motorTaskMainFastStep(&oProp)/initiateOffsetNulling(&oProp) ==
  state MainLoopFunctions
    state initiateOffsetNulling [parallel]
      settings: executionOrder=2
      state Disabled
      state Initiate
        entry:
        //We can only do this if idle
        oProp.oIsr_.oState_.fOffsetIntegratorIa_ = 0.0;
        oProp.oIsr_.oState_.fOffsetIntegratorIb_ = 0.0;
        oProp.oIsr_.oState_.fOffsetIntegratorIc_ = 0.0;
        oProp.oIsr_.oState_.fOffsetIntegratorIdc_ = 0.0;
        oProp.oMot_.oState_.uiDriveState_ = 95;
      (default) -> MainLoopFunctions.initiateOffsetNulling.Disabled
      MainLoopFunctions.initiateOffsetNulling.Disabled -> Initiate : [oProp.oMot_.oIn_.uiCurrentOffsetNullingActive_ == 1 ....
          | && (oProp.oMot_.oState_.uiDriveState_ >= 99 ....
          |  || oProp.oMot_.oState_.uiDriveState_ < 102)]
      Initiate -> MainLoopFunctions.initiateOffsetNulling.Disabled : [(oProp.oMot_.oIn_.uiCurrentOffsetNullingActive_ == 0)]
    state initiateVoltageOffsetNulling [parallel]
      settings: executionOrder=1
      state Disabled
      state initiate
        entry:
        // Must do this at 50 % duty
        // Set the offsets to zero:
        fTemp = 0.5F;
        // In the future, there may be reasons to zero the offsets at duties different than 50%.
        // Set the target duty here
        oProp.oMot_.oState_.uiDriveState_ = 245;
        oProp.oMot_.oOut_.uiPwmRequestFromMain_ = 1;
        oProp.oMot_.oOut_.uiPwmDutyTicksFromMainA_ = cast((fTemp * oProp.oMot_.oParam_.fPwmPeriodTicksMainloopFloat_), uint32);
        oProp.oMot_.oOut_.uiPwmDutyTicksFromMainB_ = cast((fTemp * oProp.oMot_.oParam_.fPwmPeriodTicksMainloopFloat_), uint32);
        oProp.oMot_.oOut_.uiPwmDutyTicksFromMainC_ = cast((fTemp * oProp.oMot_.oParam_.fPwmPeriodTicksMainloopFloat_), uint32);
        oProp.oMot_.oOut_.uiEnableGateDrive_ = 0x7;
      (default) -> MainLoopFunctions.initiateVoltageOffsetNulling.Disabled
      MainLoopFunctions.initiateVoltageOffsetNulling.Disabled -> (junction 277) : [oProp.oMot_.oIn_.uiVoltageOffsetNullingActive_ == 1]
      (junction 277) -> MainLoopFunctions.initiateVoltageOffsetNulling.Disabled [order 1] : [oProp.oMot_.oState_.uiDriveState_ < 100 ...
          |  || oProp.oMot_.oState_.uiDriveState_ > 101] ...
          | // Only start if fully idle
      initiate -> MainLoopFunctions.initiateVoltageOffsetNulling.Disabled : [(oProp.oMot_.oIn_.uiVoltageOffsetNullingActive_ == 0)]
      (junction 277) -> initiate [order 2]
  (default) -> MainLoopFunctions
  data: oProp data_store_memory; fTemp local single
